simulink model "Problem_1"  (R2020b)
settings: Solver=VariableStepAuto  StartTime=0.0  StopTime=100  RelTol=1e-3
settings Model: Creator=HP  LastModifiedBy=HP
settings DataIOCC: ExternalInput=[t, sig1]  SaveFormat=Array  ReturnWorkspaceOutputs=off

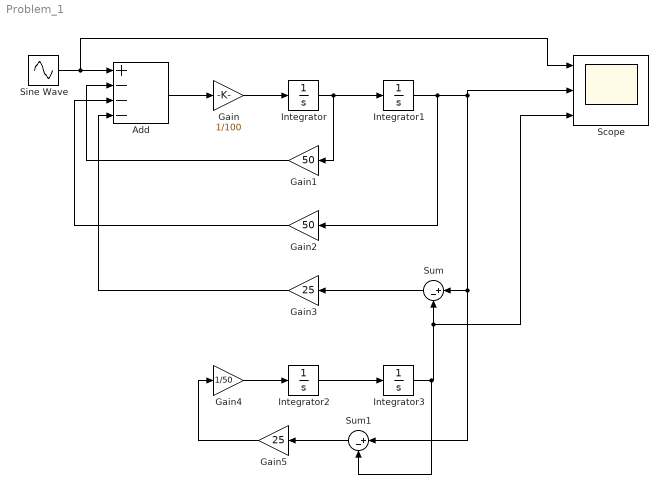
== system Problem_1 ==
  Add : Sum  Inputs=+---
  Gain : Gain  Gain=1/100
  Gain1 : Gain  Gain=50
  Gain2 : Gain  Gain=50
  Gain3 : Gain  Gain=25
  Gain4 : Gain  Gain=1/50
  Gain5 : Gain  Gain=25
  Integrator{,1..3} (4 alike) : Integrator
  Scope : Scope  NumInputPorts=3
  Sine Wave : Sin  Frequency=100  SampleTime=0
  Sum : Sum  Inputs=|+-
  Sum1 : Sum  Inputs=|+-
  wires:
  Sine Wave/1 -> Scope/1, Add/1
  Add/1 -> Gain/1
  Gain/1 -> Integrator/1
  Integrator/1 -> Integrator1/1, Gain1/1
  Integrator1/1 -> Sum1/1, Sum/1, Scope/2, Gain2/1
  Gain1/1 -> Add/2
  Gain3/1 -> Add/4
  Gain2/1 -> Add/3
  Integrator2/1 -> Integrator3/1
  Sum/1 -> Gain3/1
  Integrator3/1 -> Sum/2, Scope/3, Sum1/2
  Gain4/1 -> Integrator2/1
  Sum1/1 -> Gain5/1
  Gain5/1 -> Gain4/1
